simulink model "Rpi_send"  (R2017a)
settings: Solver=FixedStepDiscrete  StartTime=0.0  StopTime=inf  RelTol=1e-3  EnableMultiTasking=on
model workspace (MATLAB code in the model file):
  | %% define
  | imagesize = [320 240];
  | cropsize = [300 450];
  | H_start = 1;
  | W_start = 1;
  | cropsize = [imagesize(1)-H_start imagesize(2)-W_start];
  | number_local_max = 15;
  | %% molp
  | %erode_constant = strel('square',2);
  | erode_constant = 1;
  | dilation_constant = [1 1;1 1];
  | %dilation_constant = 1;
undefined symbols (not defined in the file): Rec, SDTV
libraries: hdlsllib x12, visionconversions x8, visionfilter x4, embdlinuxlib x4, simulink x4, raspberrypilib x4, visionmorphops x3, visiontransforms x3, visiongeotforms x2, visionanalysis x1, visionstatistics x1
settings Model: SimulationMode=external  ExtModeTrigDuration=100  Creator=The MathWorks, Inc.  LastModifiedBy=Pection
settings SolverCC: PositivePriorityOrder=on
settings DataIOCC: LimitDataPoints=on  SaveFormat=Array
settings OptimizationCC: ExpressionDepthLimit=2147483647  LifeSpan=Inf  MaxStackSize=64
settings DebuggingCC: UnderspecifiedInitializationDetection=Classic  MergeDetectMultiDrivingBlocksExec=none  FcnCallInpInsideContextMsg=warning  AllowSymbolicDim=off  StateNameClashWarn=warning  SFUnexpectedBacktrackingDiag=warning  SFNoUnconditionalDefaultTransitionDiag=warning  SFExecutionAtInitializationDiag=none
settings HardwareCC: ProdBitPerPointer=32  ProdBitPerSizeT=32  ProdBitPerPtrDiffT=32  ProdLargestAtomicInteger=Long  ProdLargestAtomicFloat=Double  ProdWordSize=32  ProdHWDeviceType=ARM Compatible->ARM Cortex  UseEmbeddedCoderFeatures=off  UseSimulinkCoderFeatures=off
settings ModelReferenceCC: PropagateSignalLabelsOutOfModel=off
settings RTWCC: SystemTargetFile=ert.tlc  HardwareBoard=Raspberry Pi  TLCOptions=-aInlineSetEventsForThisBaseRateFcn=TLC_FALSE -aSuppressMultiTaskScheduler=TLC_FALSE -aRateBasedStepFcn=0  TemplateMakefile=ert_default_tmf  Description=Embedded Coder  GenerateReport=on  RTWVerbose=off  Toolchain=GNU GCC Raspberry Pi  LaunchReport=on
settings CodeAppCC: ForceParamTrailComments=on  OperatorAnnotations=on  MangleLength=10  MATLABSourceComments=on
settings ERTTargetCC: MultiwordLength=2048  ERTCustomFileBanners=off  SupportContinuousTime=on  SupportNonInlinedSFcns=on  RemoveResetFunc=off  ModelStepFunctionPrototypeControlCompliant=off
settings ConfigComp: CovMetricSettings=dw  CovHtmlReporting=on  CovSaveCumulativeToWorkspaceVar=on  CovSaveSingleToWorkspaceVar=on  CovExternalEMLEnable=off

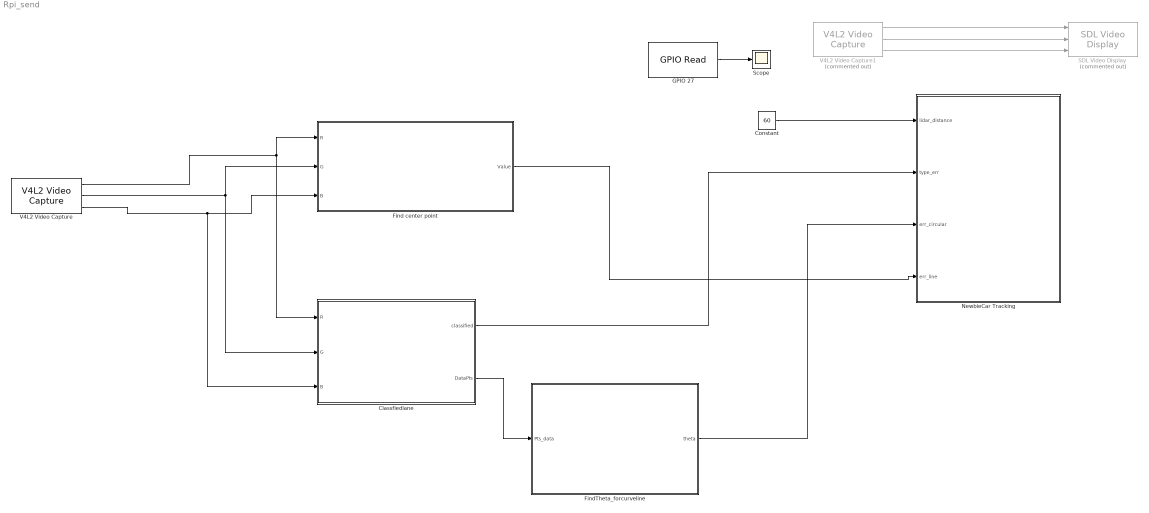
== system Rpi_send ==
  Classfiedlane : Subsystem
  Constant : Constant  Value=60
  Find center point : Subsystem
  FindTheta_forcurveline : Subsystem
  GPIO 27 : embdlinuxlib/GPIO Read  board=Model B+  gpio=27  internalResistor=Off  sampleTime=inf  direction=Input  blockPlatform=Raspberry Pi
  NewbieCar Tracking : Stateflow chart  TreatAsAtomicUnit=on
  SDL Video Display : embdlinuxlib/SDL Video Display  Commented=on  pixelFormat=RGB  pixelOrder=Planar  rowMajor=on  blockPlatform=Raspberry Pi
  Scope : Scope
  V4L2 Video Capture : embdlinuxlib/V4L2 Video Capture  m_devName='/dev/video0'  roi=[0, 0, 640, 480]  imSizeSelection=160x120  imSize=[640, 480]  pixelFormat=RGB  pixelOrder=Planar  sampleTime=0.5  simOutput=Colorbars  blockPlatform=Raspberry Pi
  V4L2 Video Capture1 : embdlinuxlib/V4L2 Video Capture  Commented=on  m_devName='/dev/video0'  roi=[0, 0, 640, 480]  imSizeSelection=640x480  imSize=[640, 480]  pixelFormat=RGB  pixelOrder=Planar  sampleTime=1/10  simOutput=Colorbars  blockPlatform=Raspberry Pi
  wires:
  V4L2 Video Capture/1 -> Classfiedlane/1("R "), Find center point/1(R)
  V4L2 Video Capture/3 -> Classfiedlane/3(B), Find center point/3(B)
  V4L2 Video Capture/2 -> Classfiedlane/2(G), Find center point/2(G)
  V4L2 Video Capture1/3 -> SDL Video Display/3
  V4L2 Video Capture1/2 -> SDL Video Display/2
  V4L2 Video Capture1/1 -> SDL Video Display/1
  GPIO 27/1 -> Scope/1
  Constant/1 -> NewbieCar Tracking/1(lidar_distance)
  Classfiedlane/2(DataPts) -> FindTheta_forcurveline/1(Pts_data)
  Find center point/1(Value) -> NewbieCar Tracking/4(err_line)
  FindTheta_forcurveline/1(theta) -> NewbieCar Tracking/3(err_circular)
  Classfiedlane/1(classified) -> NewbieCar Tracking/2(type_err)

== system Rpi_send/Classfiedlane ==
  "R " : Inport
  G : Inport  Port=2
  B : Inport  Port=3
  Subsystem : Subsystem
  "pts_selec " : MATLAB Function  TreatAsAtomicUnit=on
  classified : Outport
  DataPts : Outport  Port=2
  wires:
  Subsystem/1("Size x ") -> "pts_selec "/1(DataSizex)
  Subsystem/4("SumDataleft2 ") -> "pts_selec "/4(DataLeft2)
  Subsystem/6(sumDatamid2) -> "pts_selec "/6(DataMiddle2)
  "pts_selec "/1(classifiedLane) -> classified/1
  "R "/1 -> Subsystem/1(R)
  Subsystem/2(Size Y) -> "pts_selec "/2(DataSizey)
  Subsystem/9(DataPts) -> DataPts/1
  Subsystem/7(SumDataright1) -> "pts_selec "/7(DataRight1)
  Subsystem/8(SumDataright2) -> "pts_selec "/8(DataRight2)
  B/1 -> Subsystem/3("ฺB ")
  G/1 -> Subsystem/2(G)
  Subsystem/3(SumDataLeft1) -> "pts_selec "/3(DataLeft1)
  Subsystem/5(SumDatamid1) -> "pts_selec "/5(DataMiddle1)

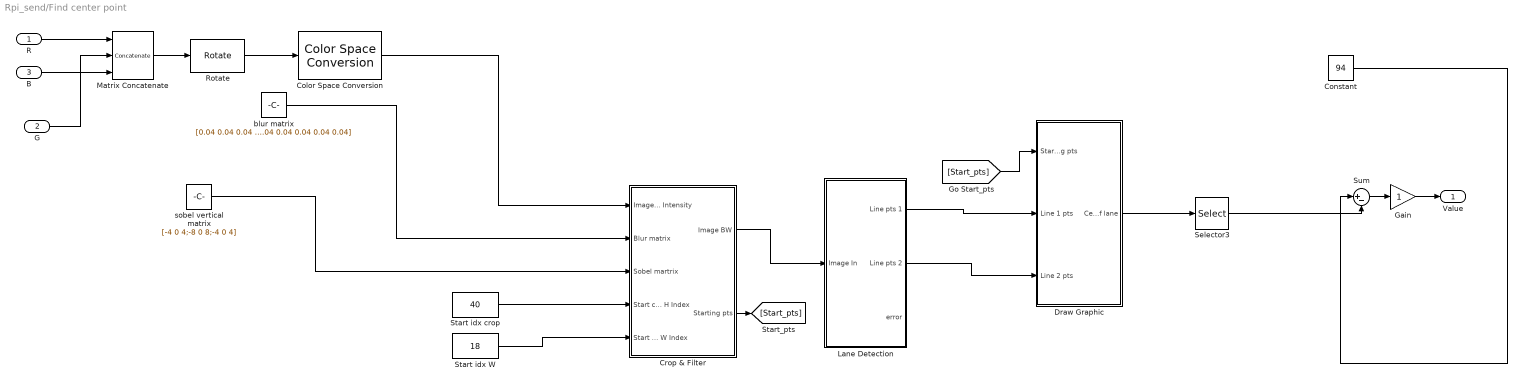
== system Rpi_send/Find center point ==
  R : Inport
  G : Inport  Port=2
  B : Inport  Port=3
  Color Space Conversion : visionconversions/Color Space  Conversion  conversion=Obsolete  conversionActive=R'G'B' to intensity  wp_str=D65  rec=Rec. 601 (SDTV)  sys=1125/60/2:1  imagePorts=One multidimensional signal
      settings: SourceProductName=Computer Vision System Toolbox
  Constant : Constant  Value=94
  Crop & Filter : Subsystem
  Draw Graphic : Subsystem
  Gain : Gain
  Lane Detection : Subsystem
  Matrix Concatenate : Concatenate  NumInputs=3  Mode=Multidimensional array  ConcatenateDimension=3
  Rotate : visiongeotforms/Rotate  outSizeR=Expanded to fit rotated input image  src_angle=Specify via dialog  unit_angle=Degrees  angle=pi/2  maxAngle=pi  dispImage=Center  method=Table lookup  fillVal=0  interpMethod=Bilinear  prodOutputMode=Binary point scaling  prodOutputWordLength=32  prodOutputFracLength=10  roundingMode=Nearest  overflowMode=on
      settings: SourceProductName=Computer Vision System Toolbox
  Selector3 : Selector  NumberOfDimensions=2  InputPortWidth=3  IndexOptions=Index vector (dialog),Index vector (dialog)  Indices=1,1  OutputSizes=1,1
  Start idx W : Constant  Value=18  OutDataTypeStr=double
  Start idx crop : Constant  Value=40  OutDataTypeStr=double
  Sum : Sum  Inputs=|+-
  blur matrix : Constant  Value=[0.04 0.04 0.04 0.04 0.04;0.04 0.04 0.04 0.04 0.04;0.04 0.04 0.04 0.04 0.04;0.04 0.04 0.04 0.04 0.04;0.04 0.04 0.04 0.04 0.04]  OutDataTypeStr=double
  sobel vertical matrix : Constant  Value=[-4 0 4;-8 0 8;-4 0 4]  OutDataTypeStr=double
  Value : Outport
  wires:
  sobel vertical matrix/1 -> Crop & Filter/3(Sobel martrix)
  Crop & Filter/1(Image BW) -> Lane Detection/1(Image In)
  R/1 -> Matrix Concatenate/1
  Color Space Conversion/1 -> Crop & Filter/1(Image Intensity)
  Lane Detection/2(Line pts 2) -> Draw Graphic/3(Line 2 pts)
  Matrix Concatenate/1 -> Rotate/1
  Start idx W/1 -> Crop & Filter/5(Start crop W Index)
  blur matrix/1 -> Crop & Filter/2(Blur matrix)
  Draw Graphic/1(Center point of lane) -> Selector3/1
  Rotate/1 -> Color Space Conversion/1
  B/1 -> Matrix Concatenate/3
  Lane Detection/1(Line pts 1) -> Draw Graphic/2(Line 1 pts)
  Crop & Filter/2(Starting pts) -> [Start_pts]
  G/1 -> Matrix Concatenate/2
  Start idx crop/1 -> Crop & Filter/4(Start crop H Index)
  [Start_pts] -> Draw Graphic/1(Starting pts)
  Constant/1 -> Sum/1
  Selector3/1 -> Sum/2
  Sum/1 -> Gain/1
  Gain/1 -> Value/1

== system Rpi_send/FindTheta_forcurveline ==
  note: gain
  Pts_data : Inport
  find point : MATLAB Function  TreatAsAtomicUnit=on
  pts_selec 2 : MATLAB Function  TreatAsAtomicUnit=on
  theta : Outport
  wires:
  Pts_data/1 -> find point/1(Datapts)
  find point/1(pts_point) -> pts_selec 2/1(point)
  pts_selec 2/1(theta) -> theta/1

== system Rpi_send/NewbieCar Tracking/circular_serial ==
  i_err1 : Inport  OutDataTypeStr=double  PortDimensions=1
  sign_err1 : Inport  Port=2  OutDataTypeStr=double  PortDimensions=1
  f : TriggerPort  TriggerType=function-call  VariantControl=Variant
      settings: CopyFcn=Stateflow.SLINSF.SimulinkMan.removeBlockPreDeleteFcn  PreDeleteFcn=Stateflow.SLINSF.SimulinkMan.unsafePredeleteFcn
  Constant : Constant  Value=0
  Constant1 : Constant  Value=0
  Package Serial Communication to freescale : Subsystem
  Serial Write : raspberrypilib/Serial Write  board=Pi 3 Model B  SCIModule_=/dev/ttyAMA0  Baudrate_=115200  Parity=None  StopBits_=1  HardwareFlowControl=None  ByteOrder=LittleEndian  OutputStatus=off  blockPlatform=RaspberryPi
      settings: SourceProductName=Simulink Support Package for Raspberry Pi Hardware  SourceProductBaseCode=RASPPI
  wires:
  sign_err1/1 -> Package Serial Communication to freescale/1(SignSteer)
  Constant/1 -> Package Serial Communication to freescale/3(SignLidar)
  i_err1/1 -> Package Serial Communication to freescale/2(SteeringAngle)
  Package Serial Communication to freescale/1(Data Output) -> Serial Write/1
  Constant1/1 -> Package Serial Communication to freescale/4(LidarAngle)

== system Rpi_send/NewbieCar Tracking/line_serial ==
  i_err : Inport  OutDataTypeStr=double  PortDimensions=1
  sign_err : Inport  Port=2  OutDataTypeStr=double  PortDimensions=1
  f : TriggerPort  TriggerType=function-call  VariantControl=Variant
      settings: CopyFcn=Stateflow.SLINSF.SimulinkMan.removeBlockPreDeleteFcn  PreDeleteFcn=Stateflow.SLINSF.SimulinkMan.unsafePredeleteFcn
  Constant : Constant  Value=0
  Constant1 : Constant  Value=0
  Package Serial Communication to freescale : Subsystem
  Serial Write : raspberrypilib/Serial Write  board=Pi 3 Model B  SCIModule_=/dev/ttyAMA0  Baudrate_=115200  Parity=None  StopBits_=1  HardwareFlowControl=None  ByteOrder=LittleEndian  OutputStatus=off  blockPlatform=RaspberryPi
      settings: SourceProductName=Simulink Support Package for Raspberry Pi Hardware  SourceProductBaseCode=RASPPI
  wires:
  Constant1/1 -> Package Serial Communication to freescale/4(LidarAngle)
  Constant/1 -> Package Serial Communication to freescale/3(SignLidar)
  Package Serial Communication to freescale/1(Data Output) -> Serial Write/1
  sign_err/1 -> Package Serial Communication to freescale/1(SignSteer)
  i_err/1 -> Package Serial Communication to freescale/2(SteeringAngle)

== system Rpi_send/NewbieCar Tracking/rapid_turn_left ==
  note: 1 is +
      | 0 is -
  lidar_angle : Inport  OutDataTypeStr=double  PortDimensions=1
  f : TriggerPort  TriggerType=function-call  VariantControl=Variant
      settings: CopyFcn=Stateflow.SLINSF.SimulinkMan.removeBlockPreDeleteFcn  PreDeleteFcn=Stateflow.SLINSF.SimulinkMan.unsafePredeleteFcn
  Package Serial Communication to freescale : Subsystem
  Serial Write : raspberrypilib/Serial Write  board=Pi 3 Model B  SCIModule_=/dev/ttyAMA0  Baudrate_=115200  Parity=None  StopBits_=1  HardwareFlowControl=None  ByteOrder=LittleEndian  OutputStatus=off  blockPlatform=RaspberryPi
      settings: SourceProductName=Simulink Support Package for Raspberry Pi Hardware  SourceProductBaseCode=RASPPI
  SignLidar : Constant  Value=0  OutDataTypeStr=uint8
  SignSteer : Constant  Value=0  OutDataTypeStr=uint8
  SteeringAngle : Constant  Value=10  OutDataTypeStr=uint8
  wires:
  Package Serial Communication to freescale/1(Data Output) -> Serial Write/1
  SignLidar/1 -> Package Serial Communication to freescale/3(SignLidar)
  SignSteer/1 -> Package Serial Communication to freescale/1(SignSteer)
  SteeringAngle/1 -> Package Serial Communication to freescale/2(SteeringAngle)
  lidar_angle/1 -> Package Serial Communication to freescale/4(LidarAngle)

== system Rpi_send/NewbieCar Tracking/rapid_turn_right ==
  lidar_angle : Inport  OutDataTypeStr=double  PortDimensions=1
  f : TriggerPort  TriggerType=function-call  VariantControl=Variant
      settings: CopyFcn=Stateflow.SLINSF.SimulinkMan.removeBlockPreDeleteFcn  PreDeleteFcn=Stateflow.SLINSF.SimulinkMan.unsafePredeleteFcn
  Package Serial Communication to freescale : Subsystem
  Serial Write : raspberrypilib/Serial Write  board=Pi 3 Model B  SCIModule_=/dev/ttyAMA0  Baudrate_=115200  Parity=None  StopBits_=1  HardwareFlowControl=None  ByteOrder=LittleEndian  OutputStatus=off  blockPlatform=RaspberryPi
      settings: SourceProductName=Simulink Support Package for Raspberry Pi Hardware  SourceProductBaseCode=RASPPI
  SignLidar : Constant  OutDataTypeStr=uint8
  SignSteer : Constant  OutDataTypeStr=uint8
  SteeringAngle : Constant  Value=10  OutDataTypeStr=uint8
  wires:
  SignLidar/1 -> Package Serial Communication to freescale/3(SignLidar)
  Package Serial Communication to freescale/1(Data Output) -> Serial Write/1
  SignSteer/1 -> Package Serial Communication to freescale/1(SignSteer)
  SteeringAngle/1 -> Package Serial Communication to freescale/2(SteeringAngle)
  lidar_angle/1 -> Package Serial Communication to freescale/4(LidarAngle)

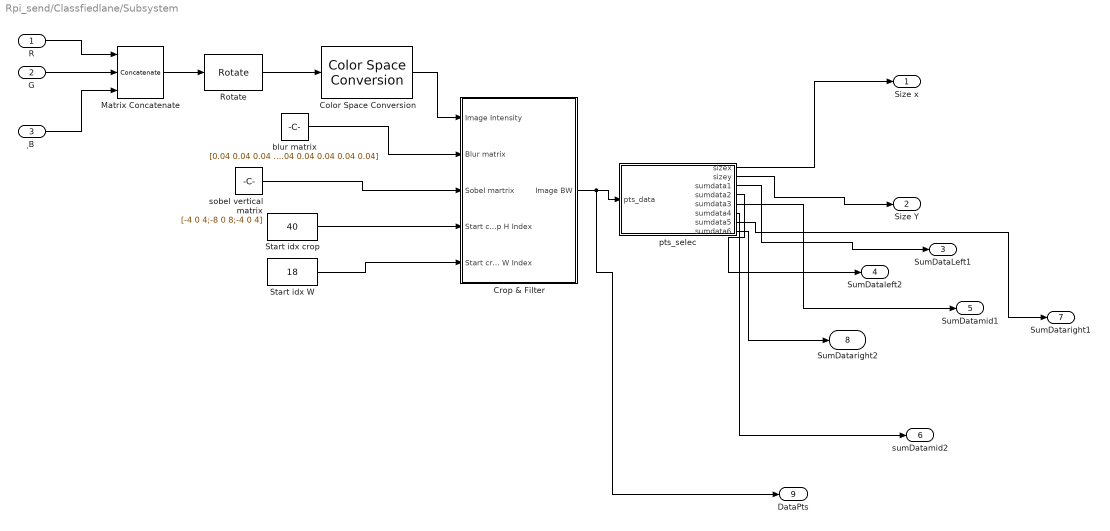
== system Rpi_send/Classfiedlane/Subsystem ==
  R : Inport
  G : Inport  Port=2
  "ฺB " : Inport  Port=3
  Color Space Conversion : visionconversions/Color Space  Conversion  conversion=Obsolete  conversionActive=R'G'B' to intensity  wp_str=D65  rec=Rec. 601 (SDTV)  sys=1125/60/2:1  imagePorts=One multidimensional signal
      settings: SourceProductName=Computer Vision System Toolbox
  Crop & Filter : Subsystem
  Matrix Concatenate : Concatenate  NumInputs=3  Mode=Multidimensional array  ConcatenateDimension=3
  Rotate : visiongeotforms/Rotate  outSizeR=Expanded to fit rotated input image  src_angle=Specify via dialog  unit_angle=Degrees  angle=pi/2  maxAngle=pi  dispImage=Center  method=Table lookup  fillVal=0  interpMethod=Bilinear  prodOutputMode=Binary point scaling  prodOutputWordLength=32  prodOutputFracLength=10  roundingMode=Nearest  overflowMode=on
      settings: SourceProductName=Computer Vision System Toolbox
  Start idx W : Constant  Value=18  OutDataTypeStr=double
  Start idx crop : Constant  Value=40  OutDataTypeStr=double
  blur matrix : Constant  Value=[0.04 0.04 0.04 0.04 0.04;0.04 0.04 0.04 0.04 0.04;0.04 0.04 0.04 0.04 0.04;0.04 0.04 0.04 0.04 0.04;0.04 0.04 0.04 0.04 0.04]  OutDataTypeStr=double
  "pts_selec " : MATLAB Function  TreatAsAtomicUnit=on
  sobel vertical matrix : Constant  Value=[-4 0 4;-8 0 8;-4 0 4]  OutDataTypeStr=double
  "Size x " : Outport
  Size Y : Outport  Port=2
  SumDataLeft1 : Outport  Port=3
  "SumDataleft2 " : Outport  Port=4
  SumDatamid1 : Outport  Port=5
  sumDatamid2 : Outport  Port=6
  SumDataright1 : Outport  Port=7
  SumDataright2 : Outport  Port=8
  DataPts : Outport  Port=9
  wires:
  G/1 -> Matrix Concatenate/2
  "ฺB "/1 -> Matrix Concatenate/3
  Start idx W/1 -> Crop & Filter/5(Start crop W Index)
  Color Space Conversion/1 -> Crop & Filter/1(Image Intensity)
  Matrix Concatenate/1 -> Rotate/1
  "pts_selec "/2(sizey) -> Size Y/1
  sobel vertical matrix/1 -> Crop & Filter/3(Sobel martrix)
  "pts_selec "/1(sizex) -> "Size x "/1
  blur matrix/1 -> Crop & Filter/2(Blur matrix)
  "pts_selec "/3(sumdata1) -> SumDataLeft1/1
  Start idx crop/1 -> Crop & Filter/4(Start crop H Index)
  R/1 -> Matrix Concatenate/1
  Rotate/1 -> Color Space Conversion/1
  "pts_selec "/8(sumdata6) -> SumDataright2/1
  "pts_selec "/6(sumdata4) -> sumDatamid2/1
  "pts_selec "/5(sumdata3) -> SumDatamid1/1
  "pts_selec "/4(sumdata2) -> "SumDataleft2 "/1
  "pts_selec "/7(sumdata5) -> SumDataright1/1
  Crop & Filter/1(Image BW) -> DataPts/1, "pts_selec "/1(pts_data)

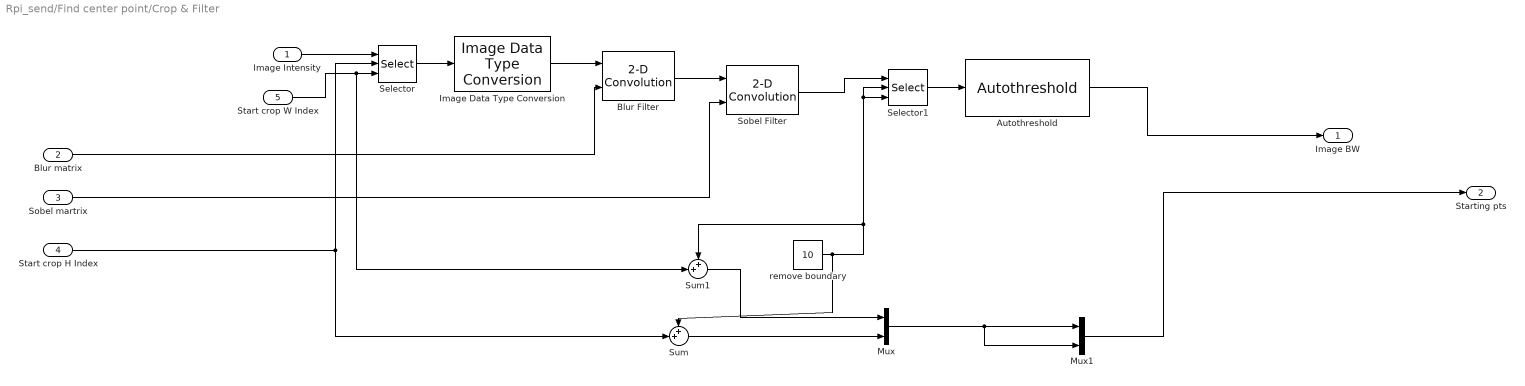
== system Rpi_send/Find center point/Crop & Filter ==
  Image Intensity : Inport
  Blur matrix : Inport  Port=2
  Sobel martrix : Inport  Port=3
  Start crop H Index : Inport  Port=4
  Start crop W Index : Inport  Port=5
  Autothreshold : visionconversions/Autothreshold  operator=>  threshOut=off  effMetricOut=off  userDefinedRange=off  umin=0  umax=255  outOfRngOpt=Warn and saturate  scaleThreshold=off  scaleFactor=1  P1Mode=Specify word length  P1WordLength=32  P1FracLength=30  P2Mode=Specify word length  P2WordLength=32  P2FracLength=22  P3Mode=Specify word length  P3WordLength=32  P3FracLength=14  P4Mode=Binary point scaling  P4WordLength=32  P4FracLength=15  Q1Mode=Specify word length  Q1WordLength=32  Q1FracLength=16  EMMode=Specify word length  EMWordLength=16  EMFracLength=14  roundingMode=Floor  overflowMode=off
      settings: SourceProductName=Computer Vision System Toolbox  SourceProductBaseCode=VP
  Blur Filter : visionfilter/2-D Convolution  outSize=Full  normalize=off  outputMode=Binary point scaling  outputWordLength=32  outputFracLength=12  prodOutputMode=Binary point scaling  prodOutputWordLength=32  prodOutputFracLength=10  roundingMode=Floor  overflowMode=off
      settings: SourceProductName=Computer Vision System Toolbox  SourceProductBaseCode=VP
  Image Data Type Conversion : visionconversions/Image Data Type Conversion  outDT=double  isSigned=on  wordLen=16  numFracBits=0
      settings: SourceProductName=Computer Vision System Toolbox  SourceProductBaseCode=VP
  Mux : Mux  Inputs=2
  Mux1 : Mux  Inputs=2
  Selector : Selector  NumberOfDimensions=2  InputPortWidth=3  IndexOptions=Starting index (port),Starting index (port)  Indices=220,1  OutputSizes=60,160
  Selector1 : Selector  NumberOfDimensions=2  InputPortWidth=3  IndexOptions=Starting index (port),Starting index (port)  Indices=10,10  OutputSizes=50,150
  Sobel Filter : visionfilter/2-D Convolution  outSize=Full  normalize=off  outputMode=Binary point scaling  outputWordLength=32  outputFracLength=12  prodOutputMode=Binary point scaling  prodOutputWordLength=32  prodOutputFracLength=10  roundingMode=Floor  overflowMode=off
      settings: SourceProductName=Computer Vision System Toolbox  SourceProductBaseCode=VP
  Sum : Sum  Inputs=++|
  Sum1 : Sum  Inputs=++|
  remove boundary : Constant  Value=10  OutDataTypeStr=double
  Image BW : Outport
  Starting pts : Outport  Port=2
  wires:
  Selector/1 -> Image Data Type Conversion/1
  Mux/1 -> Mux1/2, Mux1/1
  Mux1/1 -> Starting pts/1
  Sum/1 -> Mux/2
  Start crop H Index/1 -> Selector/2, Sum/2
  Sobel martrix/1 -> Sobel Filter/2
  Blur matrix/1 -> Blur Filter/2
  Blur Filter/1 -> Sobel Filter/1
  Sobel Filter/1 -> Selector1/1
  Selector1/1 -> Autothreshold/1
  Image Data Type Conversion/1 -> Blur Filter/1
  Image Intensity/1 -> Selector/1
  remove boundary/1 -> Sum1/1, Selector1/3, Selector1/2, Sum/1
  Autothreshold/1 -> Image BW/1
  Start crop W Index/1 -> Sum1/2, Selector/3
  Sum1/1 -> Mux/1

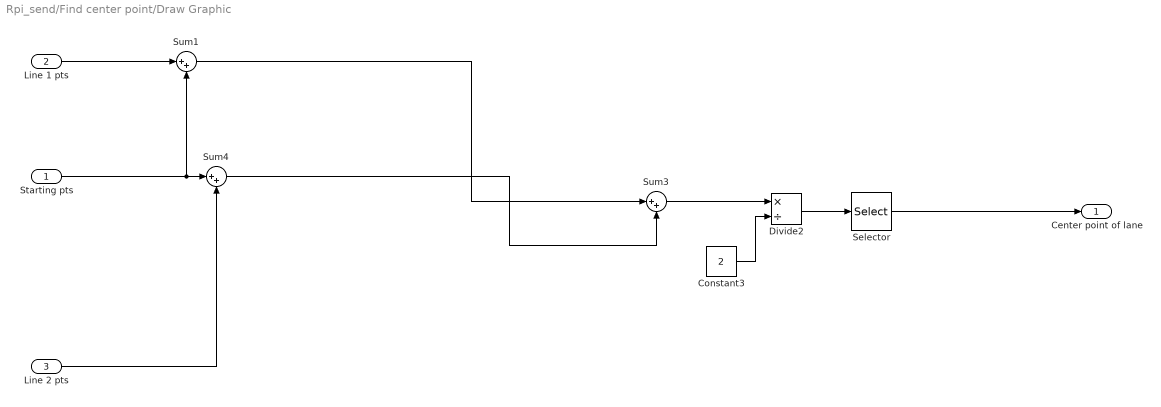
== system Rpi_send/Find center point/Draw Graphic ==
  Starting pts : Inport
  Line 1 pts : Inport  Port=2
  Line 2 pts : Inport  Port=3
  Constant3 : Constant  Value=2
  Divide2 : Product  Inputs=*/
  Selector : Selector  NumberOfDimensions=2  InputPortWidth=3  IndexOptions=Index vector (dialog),Index vector (dialog)  Indices=1,[3 4]  OutputSizes=1,1
  Sum1 : Sum  Inputs=|++
  Sum3 : Sum  Inputs=|++
  Sum4 : Sum  Inputs=|++
  Center point of lane : Outport
  wires:
  Sum1/1 -> Sum3/1
  Sum4/1 -> Sum3/2
  Sum3/1 -> Divide2/1
  Constant3/1 -> Divide2/2
  Divide2/1 -> Selector/1
  Selector/1 -> Center point of lane/1
  Line 2 pts/1 -> Sum4/2
  Starting pts/1 -> Sum4/1, Sum1/2
  Line 1 pts/1 -> Sum1/1

== system Rpi_send/Find center point/Lane Detection ==
  Image In : Inport
  Edge Detection : Subsystem
  Hough Line : Subsystem
  Image Data Type Conversion : visionconversions/Image Data Type Conversion  outDT=double  isSigned=on  wordLen=16  numFracBits=0
      settings: SourceProductName=Computer Vision System Toolbox  SourceProductBaseCode=VP
  Line pts 1 : Outport
  Line pts 2 : Outport  Port=2
  error : Outport  Port=3
  wires:
  Image Data Type Conversion/1 -> Edge Detection/1("Image ")
  Image In/1 -> Image Data Type Conversion/1
  Hough Line/1(error) -> error/1
  Edge Detection/2(Image Edge BW) -> Hough Line/1(Image BW), Hough Line/2(Image Ref)
  Hough Line/2(Line 1 pts) -> Line pts 1/1
  Hough Line/3(Line 2 pts) -> Line pts 2/1

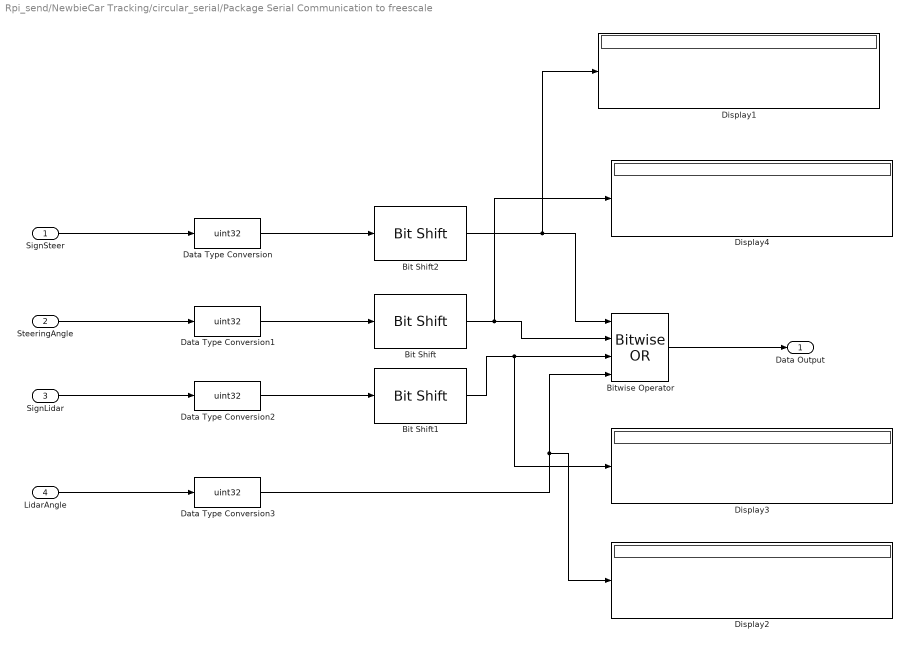
== system Rpi_send/NewbieCar Tracking/circular_serial/Package Serial Communication to freescale ==
  SignSteer : Inport
  SteeringAngle : Inport  Port=2
  SignLidar : Inport  Port=3
  LidarAngle : Inport  Port=4
  Bit Shift : hdlsllib/HDL Operations/Bit Shift  mode=Shift Left Logical  N=16
      settings: SourceProductName=HDL Coder  SourceProductBaseCode=HD
  Bit Shift1 : hdlsllib/HDL Operations/Bit Shift  mode=Shift Left Logical  N=8
      settings: SourceProductName=HDL Coder  SourceProductBaseCode=HD
  Bit Shift2 : hdlsllib/HDL Operations/Bit Shift  mode=Shift Left Logical  N=24
      settings: SourceProductName=HDL Coder  SourceProductBaseCode=HD
  Bitwise Operator : simulink/Logic and Bit Operations/Bitwise Operator  logicop=OR  UseBitMask=off  NumInputPorts=4  BitMask=bin2dec('11011001')  BitMaskRealWorld=Stored Integer
  Data Type Conversion{,1..3} (4 alike) : DataTypeConversion  OutDataTypeStr=uint32
  Display{1..4} (4 alike) : Display
      settings: Format=binary (Stored Integer)
  Data Output : Outport
  wires:
  Data Type Conversion2/1 -> Bit Shift1/1
  Bitwise Operator/1 -> Data Output/1
  Bit Shift1/1 -> Bitwise Operator/3, Display3/1
  SignLidar/1 -> Data Type Conversion2/1
  LidarAngle/1 -> Data Type Conversion3/1
  Bit Shift/1 -> Bitwise Operator/2, Display4/1
  SignSteer/1 -> Data Type Conversion/1
  Bit Shift2/1 -> Bitwise Operator/1, Display1/1
  SteeringAngle/1 -> Data Type Conversion1/1
  Data Type Conversion3/1 -> Bitwise Operator/4, Display2/1
  Data Type Conversion/1 -> Bit Shift2/1
  Data Type Conversion1/1 -> Bit Shift/1

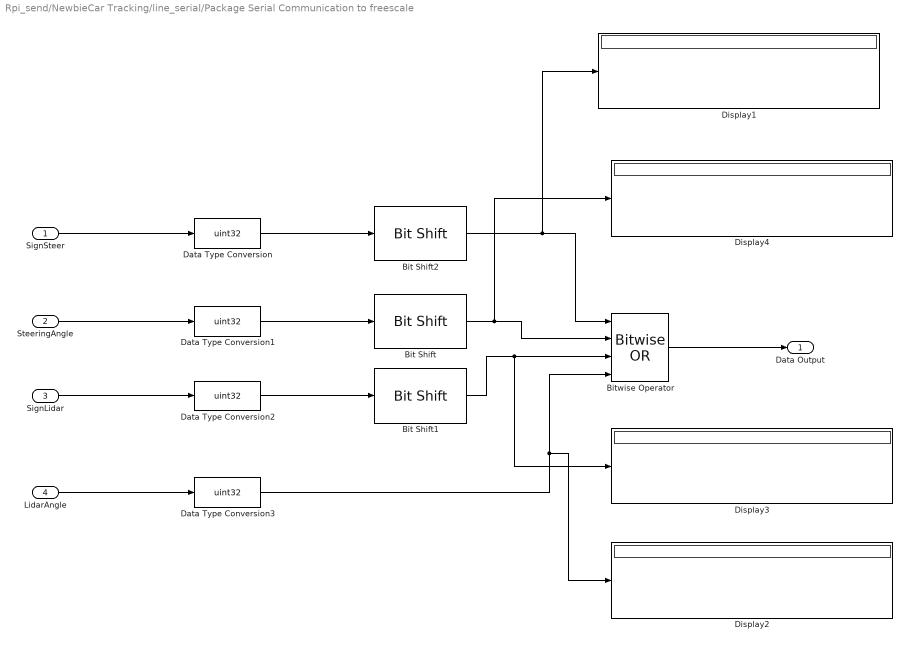
== system Rpi_send/NewbieCar Tracking/line_serial/Package Serial Communication to freescale ==
  SignSteer : Inport
  SteeringAngle : Inport  Port=2
  SignLidar : Inport  Port=3
  LidarAngle : Inport  Port=4
  Bit Shift : hdlsllib/HDL Operations/Bit Shift  mode=Shift Left Logical  N=16
      settings: SourceProductName=HDL Coder  SourceProductBaseCode=HD
  Bit Shift1 : hdlsllib/HDL Operations/Bit Shift  mode=Shift Left Logical  N=8
      settings: SourceProductName=HDL Coder  SourceProductBaseCode=HD
  Bit Shift2 : hdlsllib/HDL Operations/Bit Shift  mode=Shift Left Logical  N=24
      settings: SourceProductName=HDL Coder  SourceProductBaseCode=HD
  Bitwise Operator : simulink/Logic and Bit Operations/Bitwise Operator  logicop=OR  UseBitMask=off  NumInputPorts=4  BitMask=bin2dec('11011001')  BitMaskRealWorld=Stored Integer
  Data Type Conversion{,1..3} (4 alike) : DataTypeConversion  OutDataTypeStr=uint32
  Display{1..4} (4 alike) : Display
      settings: Format=binary (Stored Integer)
  Data Output : Outport
  wires:
  Data Type Conversion2/1 -> Bit Shift1/1
  Bitwise Operator/1 -> Data Output/1
  Bit Shift1/1 -> Bitwise Operator/3, Display3/1
  SignLidar/1 -> Data Type Conversion2/1
  LidarAngle/1 -> Data Type Conversion3/1
  Bit Shift/1 -> Bitwise Operator/2, Display4/1
  SignSteer/1 -> Data Type Conversion/1
  Bit Shift2/1 -> Bitwise Operator/1, Display1/1
  SteeringAngle/1 -> Data Type Conversion1/1
  Data Type Conversion3/1 -> Bitwise Operator/4, Display2/1
  Data Type Conversion/1 -> Bit Shift2/1
  Data Type Conversion1/1 -> Bit Shift/1

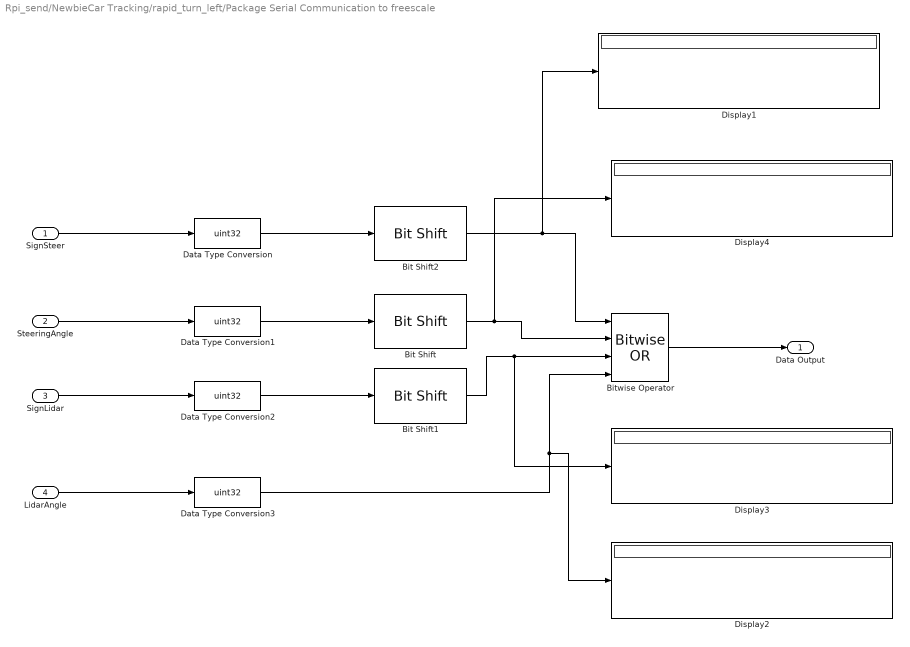
== system Rpi_send/NewbieCar Tracking/rapid_turn_left/Package Serial Communication to freescale ==
  SignSteer : Inport
  SteeringAngle : Inport  Port=2
  SignLidar : Inport  Port=3
  LidarAngle : Inport  Port=4
  Bit Shift : hdlsllib/HDL Operations/Bit Shift  mode=Shift Left Logical  N=16
      settings: SourceProductName=HDL Coder  SourceProductBaseCode=HD
  Bit Shift1 : hdlsllib/HDL Operations/Bit Shift  mode=Shift Left Logical  N=8
      settings: SourceProductName=HDL Coder  SourceProductBaseCode=HD
  Bit Shift2 : hdlsllib/HDL Operations/Bit Shift  mode=Shift Left Logical  N=24
      settings: SourceProductName=HDL Coder  SourceProductBaseCode=HD
  Bitwise Operator : simulink/Logic and Bit Operations/Bitwise Operator  logicop=OR  UseBitMask=off  NumInputPorts=4  BitMask=bin2dec('11011001')  BitMaskRealWorld=Stored Integer
  Data Type Conversion{,1..3} (4 alike) : DataTypeConversion  OutDataTypeStr=uint32
  Display{1..4} (4 alike) : Display
      settings: Format=binary (Stored Integer)
  Data Output : Outport
  wires:
  Data Type Conversion2/1 -> Bit Shift1/1
  Bitwise Operator/1 -> Data Output/1
  Bit Shift1/1 -> Bitwise Operator/3, Display3/1
  SignLidar/1 -> Data Type Conversion2/1
  LidarAngle/1 -> Data Type Conversion3/1
  Bit Shift/1 -> Bitwise Operator/2, Display4/1
  SignSteer/1 -> Data Type Conversion/1
  Bit Shift2/1 -> Bitwise Operator/1, Display1/1
  SteeringAngle/1 -> Data Type Conversion1/1
  Data Type Conversion3/1 -> Bitwise Operator/4, Display2/1
  Data Type Conversion/1 -> Bit Shift2/1
  Data Type Conversion1/1 -> Bit Shift/1

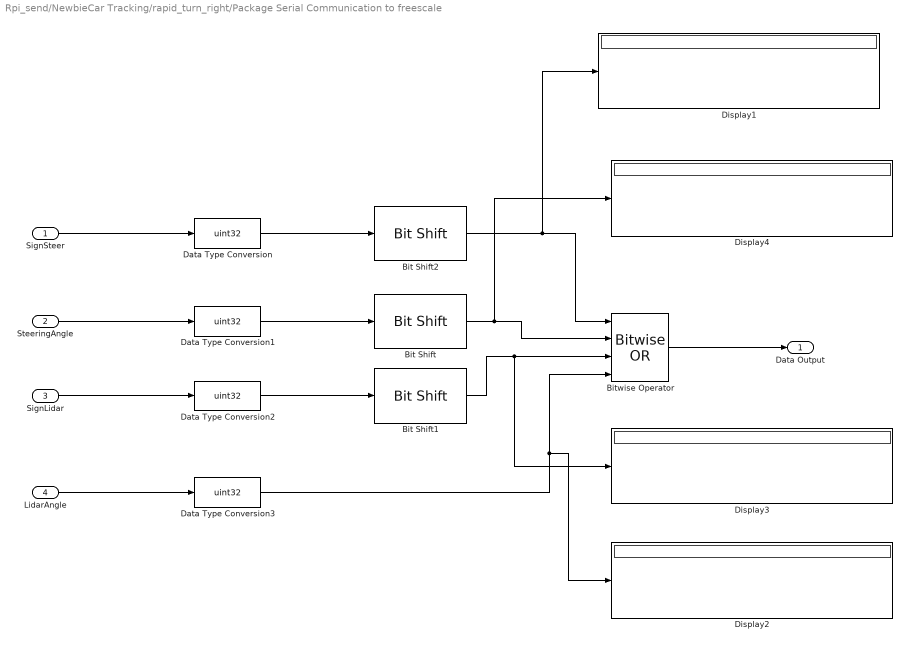
== system Rpi_send/NewbieCar Tracking/rapid_turn_right/Package Serial Communication to freescale ==
  SignSteer : Inport
  SteeringAngle : Inport  Port=2
  SignLidar : Inport  Port=3
  LidarAngle : Inport  Port=4
  Bit Shift : hdlsllib/HDL Operations/Bit Shift  mode=Shift Left Logical  N=16
      settings: SourceProductName=HDL Coder  SourceProductBaseCode=HD
  Bit Shift1 : hdlsllib/HDL Operations/Bit Shift  mode=Shift Left Logical  N=8
      settings: SourceProductName=HDL Coder  SourceProductBaseCode=HD
  Bit Shift2 : hdlsllib/HDL Operations/Bit Shift  mode=Shift Left Logical  N=24
      settings: SourceProductName=HDL Coder  SourceProductBaseCode=HD
  Bitwise Operator : simulink/Logic and Bit Operations/Bitwise Operator  logicop=OR  UseBitMask=off  NumInputPorts=4  BitMask=bin2dec('11011001')  BitMaskRealWorld=Stored Integer
  Data Type Conversion{,1..3} (4 alike) : DataTypeConversion  OutDataTypeStr=uint32
  Display{1..4} (4 alike) : Display
      settings: Format=binary (Stored Integer)
  Data Output : Outport
  wires:
  Data Type Conversion2/1 -> Bit Shift1/1
  Bitwise Operator/1 -> Data Output/1
  Bit Shift1/1 -> Bitwise Operator/3, Display3/1
  SignLidar/1 -> Data Type Conversion2/1
  LidarAngle/1 -> Data Type Conversion3/1
  Bit Shift/1 -> Bitwise Operator/2, Display4/1
  SignSteer/1 -> Data Type Conversion/1
  Bit Shift2/1 -> Bitwise Operator/1, Display1/1
  SteeringAngle/1 -> Data Type Conversion1/1
  Data Type Conversion3/1 -> Bitwise Operator/4, Display2/1
  Data Type Conversion/1 -> Bit Shift2/1
  Data Type Conversion1/1 -> Bit Shift/1

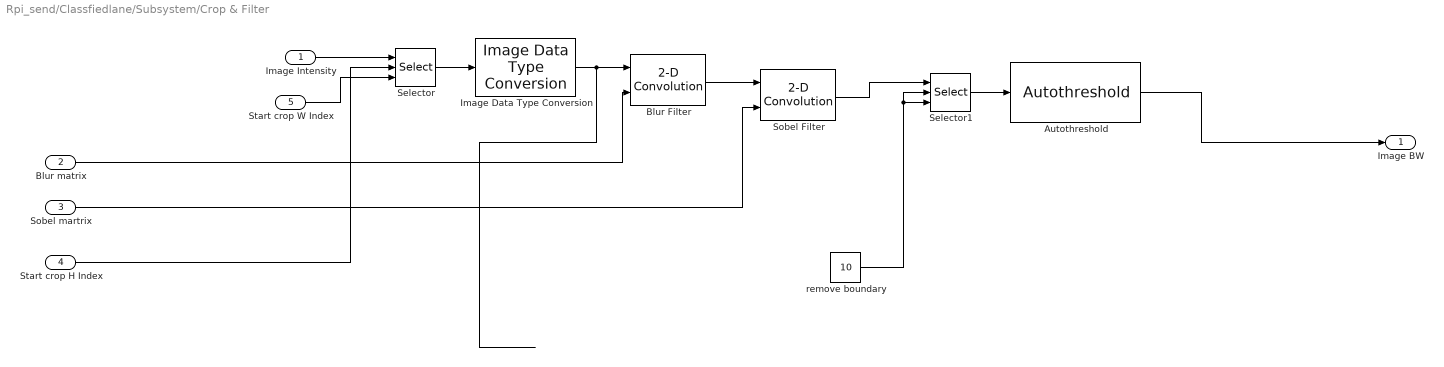
== system Rpi_send/Classfiedlane/Subsystem/Crop & Filter ==
  Image Intensity : Inport
  Blur matrix : Inport  Port=2
  Sobel martrix : Inport  Port=3
  Start crop H Index : Inport  Port=4
  Start crop W Index : Inport  Port=5
  Autothreshold : visionconversions/Autothreshold  operator=>  threshOut=off  effMetricOut=off  userDefinedRange=off  umin=0  umax=255  outOfRngOpt=Warn and saturate  scaleThreshold=off  scaleFactor=1  P1Mode=Specify word length  P1WordLength=32  P1FracLength=30  P2Mode=Specify word length  P2WordLength=32  P2FracLength=22  P3Mode=Specify word length  P3WordLength=32  P3FracLength=14  P4Mode=Binary point scaling  P4WordLength=32  P4FracLength=15  Q1Mode=Specify word length  Q1WordLength=32  Q1FracLength=16  EMMode=Specify word length  EMWordLength=16  EMFracLength=14  roundingMode=Floor  overflowMode=off
      settings: SourceProductName=Computer Vision System Toolbox  SourceProductBaseCode=VP
  Blur Filter : visionfilter/2-D Convolution  outSize=Full  normalize=off  outputMode=Binary point scaling  outputWordLength=32  outputFracLength=12  prodOutputMode=Binary point scaling  prodOutputWordLength=32  prodOutputFracLength=10  roundingMode=Floor  overflowMode=off
      settings: SourceProductName=Computer Vision System Toolbox  SourceProductBaseCode=VP
  Image Data Type Conversion : visionconversions/Image Data Type Conversion  outDT=double  isSigned=on  wordLen=16  numFracBits=0
      settings: SourceProductName=Computer Vision System Toolbox  SourceProductBaseCode=VP
  Selector : Selector  NumberOfDimensions=2  InputPortWidth=3  IndexOptions=Starting index (port),Starting index (port)  Indices=220,1  OutputSizes=60,140
  Selector1 : Selector  NumberOfDimensions=2  InputPortWidth=3  IndexOptions=Starting index (port),Starting index (port)  Indices=10,10  OutputSizes=50,130
  Sobel Filter : visionfilter/2-D Convolution  outSize=Full  normalize=off  outputMode=Binary point scaling  outputWordLength=32  outputFracLength=12  prodOutputMode=Binary point scaling  prodOutputWordLength=32  prodOutputFracLength=10  roundingMode=Floor  overflowMode=off
      settings: SourceProductName=Computer Vision System Toolbox  SourceProductBaseCode=VP
  remove boundary : Constant  Value=10  OutDataTypeStr=double
  Image BW : Outport
  wires:
  Selector/1 -> Image Data Type Conversion/1
  Start crop H Index/1 -> Selector/2
  Sobel martrix/1 -> Sobel Filter/2
  Blur matrix/1 -> Blur Filter/2
  Blur Filter/1 -> Sobel Filter/1
  Selector1/1 -> Autothreshold/1
  Image Data Type Conversion/1 -> Blur Filter/1
  Image Intensity/1 -> Selector/1
  remove boundary/1 -> Selector1/3, Selector1/2
  Autothreshold/1 -> Image BW/1
  Start crop W Index/1 -> Selector/3
  Sobel Filter/1 -> Selector1/1

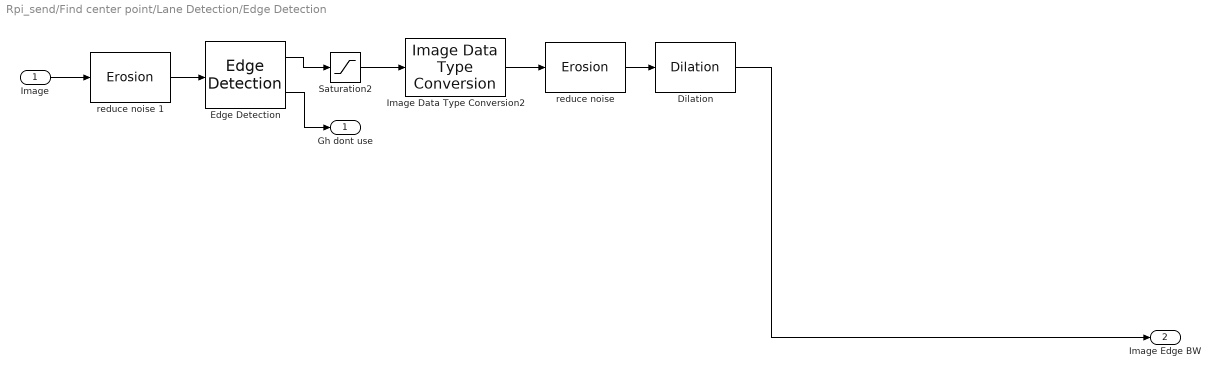
== system Rpi_send/Find center point/Lane Detection/Edge Detection ==
  "Image " : Inport
  Dilation : visionmorphops/Dilation  nhoodsrc=Specify via dialog  strel=dilation_constant
      settings: SourceProductName=Computer Vision System Toolbox  SourceProductBaseCode=VP
  Edge Detection : visionanalysis/Edge Detection  method=Sobel  outputType=Gradient components  userDefinedThreshold=on  thresholdSource=Specify via dialog  threshold=1  thresholdTuning=1  edgeThinning=on  threshold_canny=[0.25 0.60]  autoPercent=70  sigma=1  prodOutputMode=Binary point scaling  prodOutputWordLength=32  prodOutputFracLength=8  roundingMode=Floor  overflowMode=off
      settings: SourceProductName=Computer Vision System Toolbox  SourceProductBaseCode=VP
  Image Data Type Conversion2 : visionconversions/Image Data Type Conversion  outDT=boolean  isSigned=on  wordLen=16  numFracBits=0
      settings: SourceProductName=Computer Vision System Toolbox  SourceProductBaseCode=VP
  Saturation2 : Saturate  UpperLimit=1  LowerLimit=0
  "reduce noise " : visionmorphops/Erosion  nhoodsrc=Specify via dialog  strel=erode_constant
      settings: SourceProductName=Computer Vision System Toolbox  SourceProductBaseCode=VP
  reduce noise 1 : visionmorphops/Erosion  nhoodsrc=Specify via dialog  strel=erode_constant
      settings: SourceProductName=Computer Vision System Toolbox  SourceProductBaseCode=VP
  Gh dont use : Outport
  Image Edge BW : Outport  Port=2
  wires:
  Edge Detection/1 -> Saturation2/1
  "reduce noise "/1 -> Dilation/1
  Saturation2/1 -> Image Data Type Conversion2/1
  Image Data Type Conversion2/1 -> "reduce noise "/1
  reduce noise 1/1 -> Edge Detection/1
  Edge Detection/2 -> Gh dont use/1
  "Image "/1 -> reduce noise 1/1
  Dilation/1 -> Image Edge BW/1

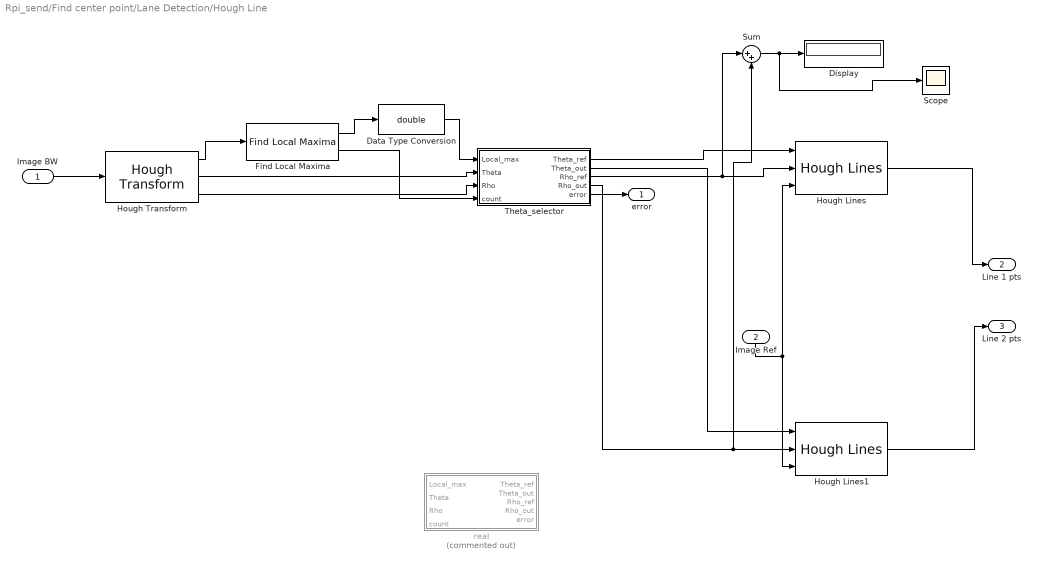
== system Rpi_send/Find center point/Lane Detection/Hough Line ==
  Image BW : Inport
  Image Ref : Inport  Port=2
  Data Type Conversion : DataTypeConversion  OutDataTypeStr=double
  Display : Display
  Find Local Maxima : visionstatistics/Find Local Maxima  num_peaks=number_local_max  nhood_size=[5 7]  src_thresh=Obsolete9b  src_thresh_inuse=Specify via dialog  threshold=10  inputIsHough=off  dt_peak=uint32  isOutVarDim=off  dt_count=uint32
      settings: SourceProductName=Computer Vision System Toolbox  SourceProductBaseCode=VP
  Hough Lines : visiontransforms/Hough Lines  sineCompMethod=Trigonometric function  thetaRes=pi/180  firstCoeffMode=Specify word length  firstCoeffWordLength=16  firstCoeffFracLength=15  prodOutputMode=Binary point scaling  prodOutputWordLength=32  prodOutputFracLength=16  roundingMode=Nearest  overflowMode=on
      settings: SourceProductName=Computer Vision System Toolbox  SourceProductBaseCode=VP
  Hough Lines1 : visiontransforms/Hough Lines  sineCompMethod=Trigonometric function  thetaRes=pi/180  firstCoeffMode=Specify word length  firstCoeffWordLength=16  firstCoeffFracLength=15  prodOutputMode=Binary point scaling  prodOutputWordLength=32  prodOutputFracLength=16  roundingMode=Nearest  overflowMode=on
      settings: SourceProductName=Computer Vision System Toolbox  SourceProductBaseCode=VP
  Hough Transform : visiontransforms/Hough Transform  theta_res=pi/360  rho_res=1  out_theta_rho=on  outdtmode=double  firstCoeffMode=Binary point scaling  firstCoeffWordLength=16  firstCoeffFracLength=14  secondCoeffMode=Binary point scaling  secondCoeffWordLength=32  secondCoeffFracLength=16  outputMode=Binary point scaling  outputWordLength=16  outputFracLength=0  accumMode=Binary point scaling  accumWordLength=32  accumFracLength=20  prodOutputMode=Binary point scaling  prodOutputWordLength=32  prodOutputFracLength=20  memoryMode=Binary point scaling  memoryWordLength=32  memoryFracLength=16  roundingMode=Nearest  overflowMode=on
      settings: SourceProductName=Computer Vision System Toolbox  SourceProductBaseCode=VP
  Scope : Scope
  Sum : Sum  Inputs=|++
  Theta_selector : MATLAB Function  TreatAsAtomicUnit=on
  real : MATLAB Function  Commented=on  TreatAsAtomicUnit=on
  error : Outport
  Line 1 pts : Outport  Port=2
  Line 2 pts : Outport  Port=3
  wires:
  Find Local Maxima/2 -> Theta_selector/4(count)
  Image Ref/1 -> Hough Lines/3, Hough Lines1/3
  Image BW/1 -> Hough Transform/1
  Theta_selector/1(Theta_ref) -> Hough Lines/1
  Find Local Maxima/1 -> Data Type Conversion/1
  Theta_selector/4(Rho_out) -> Hough Lines1/2, Sum/2
  Data Type Conversion/1 -> Theta_selector/1(Local_max)
  Theta_selector/5(error) -> error/1
  Hough Transform/2 -> Theta_selector/2(Theta)
  Hough Transform/3 -> Theta_selector/3(Rho)
  Theta_selector/3(Rho_ref) -> Sum/1, Hough Lines/2
  Theta_selector/2(Theta_out) -> Hough Lines1/1
  Hough Transform/1 -> Find Local Maxima/1
  Hough Lines/1 -> Line 1 pts/1
  Hough Lines1/1 -> Line 2 pts/1
  Sum/1 -> Scope/1, Display/1

== stateflow chart Rpi_send/NewbieCar Tracking ==
  state SettingUp
    entry:lane = 0; % zero left, one right
  state TrackingLine
    state Init_Tracking
      entry: exit_lidar_state = 0;
    state Circular_Tracking
      during:
      if(err_circular <= 0)
      circular_serial(-1*err_circular,0);
      elseif(err_circular > 0)
      circular_serial(err_circular,1);
      end
    state Linear_Tracking
      during:
      if(err_line <= 0)
      line_serial(-1*err_line,0);
      elseif(err_line > 0)
      line_serial(err_line,1);
      end
    (default) -> Init_Tracking
    Init_Tracking -> Linear_Tracking [order 1] : [type_err == 0]
    Init_Tracking -> Circular_Tracking [order 2] : [type_err ==1]
    Linear_Tracking -> Circular_Tracking : [type_err == 1]
    Circular_Tracking -> Linear_Tracking : [type_err == 0]
  state LIDAR_STATE
    state Turn_and_tracking
      during:
      if(err_line < 0)
      line_serial(err_line,0);
      elseif(err_line > 0)
      line_serial(err_line,1);
      end
    state Rapid_turn_to_other_lane
      during:
      if lane == 0
      rapid_turn_right(20);
      elseif lane == 1
      rapid_turn_left(20);
      end
      exit:
      if lane == 0
      lane = 1;
      elseif lane == 1
      lane = 0;
      end
    state Back_to_the_lane
      during:
      if lane == 0
      rapid_turn_right(0);
      elseif lane == 1
      rapid_turn_left(0);
      end
      exit:
      if lane == 0
      lane = 1;
      elseif lane == 1
      lane = 0;
      end
    state exit_lidar
      entry: exit_lidar_state = 1;
    (default) -> Rapid_turn_to_other_lane
    Rapid_turn_to_other_lane -> Turn_and_tracking : [after(2,sec)]
    Turn_and_tracking -> Back_to_the_lane : [lidar_distance >40]
    Back_to_the_lane -> exit_lidar : after(2,sec)
  state line_serial(i_err,sign_err) [function]
  state circular_serial(i_err1,sign_err1) [function]
  state rapid_turn_left(lidar_angle) [function]
  state rapid_turn_right(lidar_angle) [function]
  (default) -> SettingUp
  SettingUp -> TrackingLine : [after(2,sec)]
  TrackingLine -> LIDAR_STATE : [lidar_distance <50]
  LIDAR_STATE -> TrackingLine : [exit_lidar_state == 1]
  data: i_err function_input double size=1; sign_err function_input double size=1; i_err1 function_input double size=1; sign_err1 function_input double size=1; lidar_angle function_input double size=1; lidar_angle function_input double size=1; lidar_distance input; lane local; type_err input; exit_lidar_state local; err_circular input; err_line input

== matlab function Rpi_send/Find center point/Lane Detection/Hough Line/Theta_selector ==
  data: Theta_ref output; Theta_out output; Rho_ref output; Local_max input; Theta input; Rho input; Rho_out output; error output; count input
function [Theta_ref,Theta_out,Rho_ref,Rho_out,error] = Theta_selector(Local_max,Theta,Rho,count)
[H,W] = size(Local_max);
error = 0;
mem = 100;
idx_out = 1;
%%
if count > 1
for x = 1:H
    if Theta(Local_max(x,1)) < 0
        Theta_ref = Theta(Local_max(x,1));
        Rho_ref = Rho(Local_max(x,2));
        break;
    else
    Theta_ref=Theta(Local_max(x,1));
    Rho_ref = Rho(Local_max(x,2));
    end
end

%% abs
for x = 1:H
A = abs(Theta(Local_max(x,1)) + Theta_ref);
    if A < mem
        mem = A;
        idx_out = x;
    end
end
Theta_out = Theta(Local_max(idx_out,1));
Rho_out = Rho(Local_max(idx_out,2));
%% error

if Theta_out > 1 | Theta_ref > 1
        error = 1;
end
if (Theta_out > 0 && Theta_ref > 0) | (Theta_out < 0 && Theta_ref < 0)
        error = 1;
end
else
    Theta_ref=Theta(Local_max(1,1));
    Rho_ref = Rho(Local_max(1,2));
    Theta_out=Theta(Local_max(1,1));
    Rho_out = Rho(Local_max(1,2));
end

== matlab function Rpi_send/Find center point/Lane Detection/Hough Line/real ==
  data: Theta_ref output; Theta_out output; Rho_ref output; Local_max input; Theta input; Rho input; Rho_out output; error output; count input
function [Theta_ref,Theta_out,Rho_ref,Rho_out,error] = Theta_selector(Local_max,Theta,Rho,count)
[H,W] = size(Local_max);
error = 0;
%%
if count > 1
for x = 1:H
    if Theta(Local_max(x,1)) > 0
        Theta_ref = Theta(Local_max(x,1));
        Rho_ref = Rho(Local_max(x,2));
        break;
    else
    Theta_ref=Theta(Local_max(x,1));
    Rho_ref = Rho(Local_max(x,2));
    end
end

for x = 1:H
    if Theta(Local_max(x,1)) < 0
        Theta_out = Theta(Local_max(x,1));
        Rho_out = Rho(Local_max(x,2));
        break;
    else
    Theta_out=Theta(Local_max(x,1));
    Rho_out = Rho(Local_max(x,2));
    end
end
%% error

if Theta_out > 1 | Theta_ref > 1
        error = 1;
end
if (Theta_out > 0 && Theta_ref > 0) | (Theta_out < 0 && Theta_ref < 0)
        error = 1;
end
else
    Theta_ref=Theta(Local_max(1,1));
    Rho_ref = Rho(Local_max(1,2));
    Theta_out=Theta(Local_max(1,1));
    Rho_out = Rho(Local_max(1,2));
end

== matlab function Rpi_send/Classfiedlane/Subsystem/pts_selec  ==
  data: sizex output; sizey output; sumdata1 output; sumdata2 output; sumdata3 output; pts_data input; sumdata4 output; sumdata5 output; sumdata6 output
function [sizex,sizey,sumdata1,sumdata2,sumdata3,sumdata4,sumdata5,sumdata6]  = selecdata(pts_data)
[sizex,sizey] =size(pts_data)

data1 =pts_data(25,1:20)
data2 = pts_data(25,20:40)
data3 =pts_data(25,40:60)
data4 =pts_data(25,60:80)
data5 =pts_data(25,100:120)
data6 =pts_data(25,120:end)

sumdata1 = sum(data1)
sumdata2 = sum(data2)
sumdata3 = sum(data3)
sumdata4 = sum(data4)
sumdata5 = sum(data5)
sumdata6 = sum(data6)

== matlab function Rpi_send/Classfiedlane/pts_selec  ==
  data: classifiedLane output; DataSizex input; DataSizey input; DataLeft1 input; DataLeft2 input; DataMiddle1 input; DataMiddle2 input; DataRight1 input; DataRight2 input
function classifiedLane   = selecdata(DataSizex,DataSizey,DataLeft1,DataLeft2,DataMiddle1,DataMiddle2,DataRight1,DataRight2)
classifiedLane = 10

if DataLeft1+ DataLeft2 > 5 && DataRight2+DataRight1 > 4
    classifiedLane = 0
elseif DataLeft1+ DataLeft2 > 5 && DataRight2+DataRight1 < 1
    classifiedLane = 0
elseif DataLeft1+DataLeft2+DataRight1+DataRight2+DataMiddle1+DataMiddle2 ==0
    classifiedLane =0
else 
    classifiedLane = 1
end

== matlab function Rpi_send/FindTheta_forcurveline/find point ==
  data: pts_point output; Datapts input
function pts_point = findpointx(Datapts)
pts_point = 0
for i = 1:120
    if Datapts(25,i) ==1 
        pts_point = i
        break
    end
end

== matlab function Rpi_send/FindTheta_forcurveline/pts_selec 2 ==
  data: theta output; point input
function theta = finddtheta(point)
data1 = point-20
data2 = 50-25
data3 = data1/data2
theta = atan2(data1,data2)
